simulink subsystem "CollisionDetection"  (R2024b)
settings: Solver=VariableStepAuto  StartTime=0.0  StopTime=10.0  RelTol=1e-3
undefined symbols (not defined in the file): actorProfiles, assessment
settings Model: Creator=The MathWorks, Inc.  LastModifiedBy=The MathWorks, Inc.
settings SolverCC: MaxZcPerStep=1
settings DebuggingCC: UnconnectedInputMsg=warning  UnconnectedOutputMsg=warning  UnconnectedLineMsg=warning  SubsystemReferenceDiagnosticForUnitTest=warning
settings ModelReferenceCC: EnableRefExpFcnMdlSchedulingChecks=on
settings RTWCC: GPUComputeCapability=3.5  DLArmComputeVersion=19.05

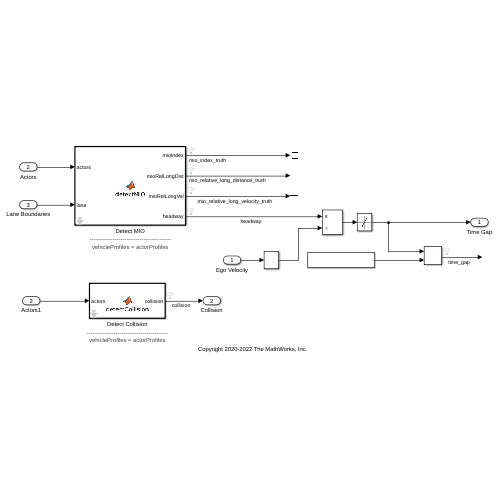
[thumbnail: Simulink's stored preview of the top-level diagram]
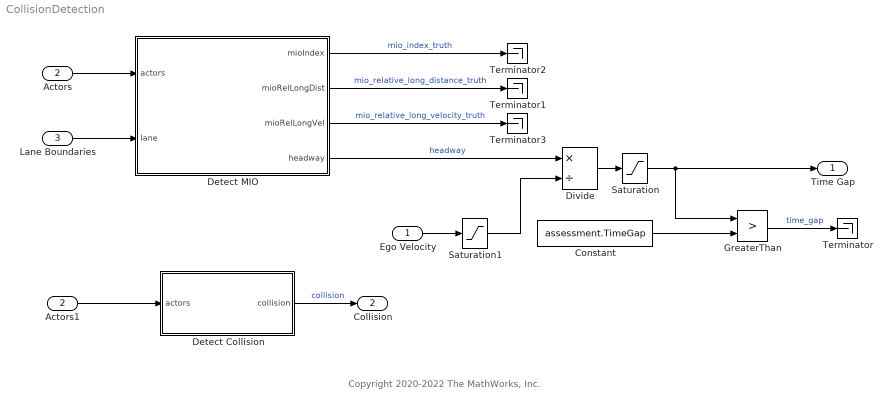
== system CollisionDetection ==
  note: Copyright 2020-2022 The MathWorks, Inc.
  Ego Velocity : Inport
  Actors : Inport  Port=2
  Lane Boundaries : Inport  Port=3
  Actors1 : InportShadow  Port=2
  Constant : Constant  Value=assessment.TimeGap
  Detect Collision : MATLAB Function  TreatAsAtomicUnit=on  mask(Detect Collision){vehicleProfiles=actorProfiles}
      mask prompts: vehicleProfiles "Vehicle profiles"
      mask help:
      | Detect collision between ego and target vehicles.
      | Vehicle profiles is expected to be the struture returned by the actorProfiles method of a drivingScenerio object.
      settings: AttributesFormatString=|
      | ------------------------------------------
      | vehicleProfiles = %<vehicleProfiles>
  Detect MIO : MATLAB Function  TreatAsAtomicUnit=on  mask(Detect Most Important Obejct (MIO)){vehicleProfiles=actorProfiles}
      mask prompts: vehicleProfiles "Vehicle profiles"
      mask help:
      | Detect most important object (MIO) in ego vehicle lane.
      | Headway to MIO takes into account the vehicel dimensions.
      | Vehicle profiles is expected to be the struture returned by the actorProfiles method of a drivingScenerio object.
      settings: AttributesFormatString=|
      | ------------------------------------------
      | vehicleProfiles = %<vehicleProfiles>
  Divide : Product  Inputs=*/
  GreaterThan : RelationalOperator  Operator=>  OutDataTypeStr=boolean  RndMeth=Simplest  InputSameDT=off
  Saturation : Saturate  UpperLimit=4  LowerLimit=0
  Saturation1 : Saturate  UpperLimit=100  LowerLimit=0.01
  Terminator{,1..3} (4 alike) : Terminator
  Time Gap : Outport
  Collision : Outport  Port=2
  wires:
  Actors/1 -> Detect MIO/1(actors)
  Lane Boundaries/1 -> Detect MIO/2(lane)
  Detect MIO/4(headway) -> Divide/1  "headway"
  Ego Velocity/1 -> Saturation1/1
  Divide/1 -> Saturation/1
  Saturation/1 -> GreaterThan/1, Time Gap/1
  Saturation1/1 -> Divide/2
  Constant/1 -> GreaterThan/2
  GreaterThan/1 -> Terminator/1  "time_gap"
  Detect MIO/2(mioRelLongDist) -> Terminator1/1  "mio_relative_long_distance_truth"
  Detect MIO/1(mioIndex) -> Terminator2/1  "mio_index_truth"
  Detect Collision/1(collision) -> Collision/1  "collision"
  Detect MIO/3(mioRelLongVel) -> Terminator3/1  "mio_relative_long_velocity_truth"
  Actors1/1 -> Detect Collision/1(actors)

== matlab function CollisionDetection/Detect Collision ==
  data: actors input; collision output; vehicleProfiles parameter
function collision = detectCollision(actors, vehicleProfiles)

% Associate on-path MATLAB function
coder.extrinsic('helperSLDetectVehicleCollision');

% Assign default value to define output data type
collision = false;

% Call on-path MATLAB function
collision = helperSLDetectVehicleCollision(actors.Actors, vehicleProfiles);

== matlab function CollisionDetection/Detect MIO ==
  data: actors input; mioIndex output; mioRelLongDist output; mioRelLongVel output; lane input; headway output; vehicleProfiles parameter
function [mioIndex,mioRelLongDist,mioRelLongVel,headway] = detectMIO(actors,lane,vehicleProfiles)

% Find the closest vehicle in ego lane
longDist = zeros(1,actors.NumActors);
for i = 1:actors.NumActors
    
    % Positions with respect to ego
    x = actors.Actors(i).Position(1);
    y = actors.Actors(i).Position(2);
    
    % Default longitudinal distance from vehicle
    longDist(i) = inf;
    
    % Check if vehicle is ahead of ego
    if x >= 0
        % Find left lane coordinates closest to vehicle position x
        [~,n] = min(abs(lane.LaneBoundaries(1).Coordinates(:,1)-x));
        yleftLane = lane.LaneBoundaries(1).Coordinates(n,2);

        % Find right lane coordinates closest to vehicle position x
        [~,n] = min(abs(lane.LaneBoundaries(2).Coordinates(:,1)-x));
        yrightLane = lane.LaneBoundaries(2).Coordinates(n,2);

        % Check if vehicle is in same lane as ego
        if (yrightLane <= y) && (y <= yleftLane)
            longDist(i) = x;
        end       
    end
end

% Minimum distance between vehicle rear axles
[minLongDist,mioIndex] = min(longDist);

if isempty(minLongDist) || isinf(minLongDist)
    mioIndex = nan;
    mioRelLongDist = inf;
    mioRelLongVel = inf;
    headway = inf;
else
    mioRelLongDist = minLongDist;
    mioRelLongVel = actors.Actors(mioIndex).Velocity(1);
    headway = headwayLongDist(minLongDist,mioIndex,vehicleProfiles);
end

end

function headway = headwayLongDist(dist,mioIndex,vehicleProfiles)
% Longitudinal headway is distance between vehicle rear axles
% reduced by distance of ego rear axle to front and 
% reduced by distance of MIO rear axle to rear

% Notes on origin offset
% - Origin offset is the relative position [x,yz] of vehicle center with 
%   respect to the rear axle
% - Distance rear axle center to vehicle center = negative of origin offset(1)

% Ego distance from rear axle to front
egoProfile = vehicleProfiles(1);
egoDistRearAxleToVehCenter = - egoProfile.OriginOffset(1);
egoDistRearAxleToFront = egoProfile.Length/2 + egoDistRearAxleToVehCenter;

% MIO distance from rear axle to rear
mioProfile = vehicleProfiles(mioIndex);
mioDistRearAxleToVehCenter = - mioProfile.OriginOffset(1);
mioDistRearAxleToRear = mioProfile.Length/2 - mioDistRearAxleToVehCenter;

% Longitudinal headway is distance from front of ego to rear of MIO
headway = dist - egoDistRearAxleToFront - mioDistRearAxleToRear;

end
